simulink model "Q4"  (R2022a)
settings: Solver=VariableStepAuto  StartTime=0.0  StopTime=2  RelTol=1e-3
undefined symbols (not defined in the file): A, B, C, K, K1, L1
settings Model: Creator=fatae  LastModifiedBy=fatae

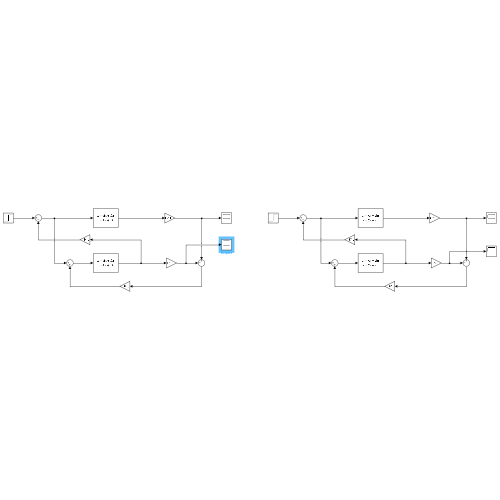
[thumbnail: Simulink's stored preview of the top-level diagram]
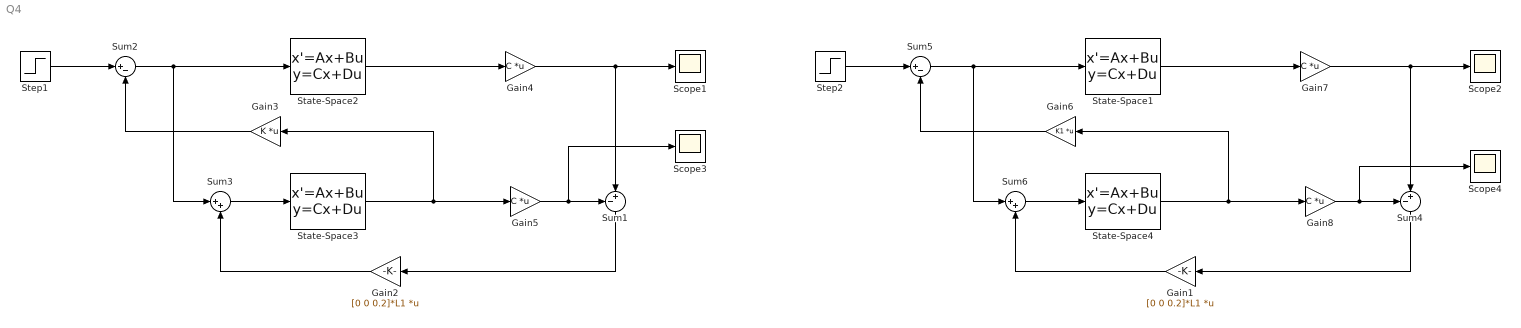
== system Q4 ==
  Gain1 : Gain  Gain=[0 0 0.2]*L1  Multiplication=Matrix(K*u)
  Gain2 : Gain  Gain=[0 0 0.2]*L1  Multiplication=Matrix(K*u)
  Gain3 : Gain  Gain=K  Multiplication=Matrix(K*u)
  Gain{4..5,7..8} (4 alike) : Gain  Gain=C  Multiplication=Matrix(K*u)
  Gain6 : Gain  Gain=K1  Multiplication=Matrix(K*u)
  Scope{1..4} (4 alike) : Scope
  State-Space{1..4} (4 alike) : StateSpace  A=A  B=B  C=[1 0 0; 0 1 0;0 0 1]  D=[0;0;0]  InitialCondition=0
  Step1 : Step  Time=0  SampleTime=0
  Step2 : Step  Time=0  SampleTime=0
  Sum1 : Sum  Inputs=-+|
  Sum2 : Sum  Inputs=|+-
  Sum3 : Sum  Inputs=|++
  Sum4 : Sum  Inputs=-+|
  Sum5 : Sum  Inputs=|+-
  Sum6 : Sum  Inputs=|++
  wires:
  State-Space2/1 -> Gain4/1
  Sum1/1 -> Gain2/1
  Step1/1 -> Sum2/1
  Gain2/1 -> Sum3/2
  Sum2/1 -> Sum3/1, State-Space2/1
  Sum3/1 -> State-Space3/1
  Gain3/1 -> Sum2/2
  State-Space3/1 -> Gain3/1, Gain5/1
  Sum4/1 -> Gain1/1
  State-Space1/1 -> Gain7/1
  Sum6/1 -> State-Space4/1
  Gain1/1 -> Sum6/2
  State-Space4/1 -> Gain6/1, Gain8/1
  Gain8/1 -> Scope4/1, Sum4/1
  Gain7/1 -> Scope2/1, Sum4/2
  Gain6/1 -> Sum5/2
  Step2/1 -> Sum5/1
  Sum5/1 -> Sum6/1, State-Space1/1
  Gain4/1 -> Scope1/1, Sum1/2
  Gain5/1 -> Scope3/1, Sum1/1
